simulink model "vehicle_dynamics_fullcar"  (R2012b)
settings: Solver=ode4  StartTime=0.0  StopTime=20  FixedStep=0.001  RelTol=1e-3
model workspace (MAT data in the model file):
  x0 = [0; 0; 0; 0; 0; 0; 0; 0; 0; 0; 0; 0; 0; 0]
undefined symbols (not defined in the file): CarBody, Suspension, Wheel
settings Model: Creator=vismso  LastModifiedBy=vikafla
settings DataIOCC: SaveFinalState=on  SignalLoggingSaveFormat=ModelDataLogs  SaveOutput=off  SaveTime=off
settings OptimizationCC: InlineParams=on
settings DebuggingCC: FcnCallInpInsideContextMsg=UseLocalSettings  StrictBusMsg=Warning
settings SFSimCC: SimParseCustomCode=off
settings GRTTargetCC: CombineOutputUpdateFcns=off  GRTInterface=on

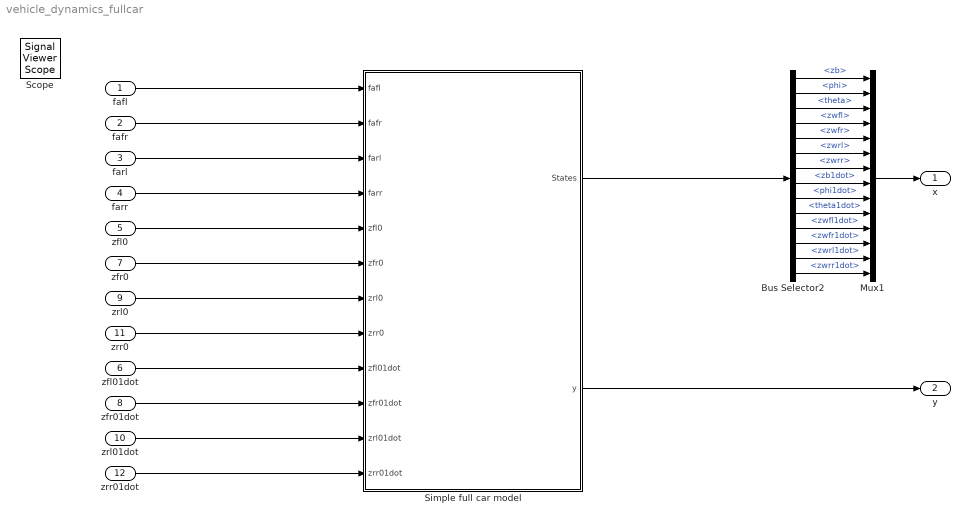
== system vehicle_dynamics_fullcar ==
  fafl : Inport
  fafr : Inport  Port=2
  farl : Inport  Port=3
  farr : Inport  Port=4
  zfl0 : Inport  Port=5
  zfl01dot : Inport  Port=6
  zfr0 : Inport  Port=7
  zfr01dot : Inport  Port=8
  zrl0 : Inport  Port=9
  zrl01dot : Inport  Port=10
  zrr0 : Inport  Port=11
  zrr01dot : Inport  Port=12
  Bus Selector2 : BusSelector  OutputSignals=zb,phi,theta,zwfl,zwfr,zwrl,zwrr,zb1dot,phi1dot,theta1dot,zwfl1dot,zwfr1dot,zwrl1dot,zwrr1dot
  Mux1 : Mux  Inputs=14
  Simple full car model : Subsystem  mask{mb=CarBody.Mass, mw=Wheel.Mass, Ibxx=CarBody.InertiaTensor(1,1), Ibyy=CarBody.InertiaTensor(2,2), lf=Suspension.MountPointFL(1), lr=-Suspension.MountPointRL(1), hf=Suspension.MountPointFL(3), hr=Suspension.MountPointRL(3), d=Suspension.MountPointFL(1)-Suspension.MountPointRL(1), tw=Suspension.MountPointFL(2)-Suspension.MountPointFR(2), r0=Wheel.UnloadedRadius, g=9.81, l0f=Suspension.SpringFreeLengthFL, l0r=Suspension.SpringFreeLengthRL, crbf=Suspension.FrontRollbarStiffness, crbr=Suspension.RearRollbarStiffness, cf=interp1(Suspension.SpringStiffnessLookUpFL(1,:).',Suspension.SpringStiffnessLookUpFL(2,:).',1,'linear','extrap'), cr=interp1(Suspension.SpringStiffnessLookUpRL(1,:).',Suspension.SpringStiffnessLookUpRL(2,:).',1,'linear','extrap'), df=5*interp1(Suspension.DamperCushioningLookUpFL(1,:).',Suspension.DamperCushioningLookUpFL(2,:).',1,'linear','extrap'), dr=7*interp1(Suspension.DamperCushioningLookUpRL(1,:).',Suspension.DamperCushioningLookUpRL(2,:).',1,'linear','extrap'), cw=Wheel.TireStiffness, dw=Wheel.TireDamping}
      mask prompts: mb "Vehicle body mass [kg]"; mw "Wheel mass [kg]"; Ibxx "Body inertia Ixx [kg m^2]"; Ibyy "Body inertia Iyy [kg m^2]"; lf "Distance from COG to front axle [m]"; lr "Distance from COG to rear axle [m]"; hf "Height of front damper mount points over COG [m]"; hr "Height of rear damper mount points over COG [m]"; d "Wheelbase [m]"; tw "Track width"; r0 "Unloaded tire radius [m]"; g "Gravity [m/s^2]"; l0f "Free length of front springs [m]"; l0r "Free length of rear springs [m]"; crbf "Front rollbar stiffness [N/m]"; crbr "Rear rollbar stiffness [N/m]"; cf "Front spring stiffness [N/m]"; cr "Rear spring stiffness [N/m]"; df "Front damper cushioning [Ns/m]"; dr "Rear damper cushioning [Ns/m]"; cw "Tire stiffness [N/m]"; dw "Tire damper cushioning [Ns/m]"
  x : Outport
  y : Outport  Port=2
  Scope : SignalViewerScope  IOType=viewer  ZoomMode=yonly  RefreshTime=0.035000
  wires:
  fafl/1 -> Simple full car model/1(fafl)
  fafr/1 -> Simple full car model/2(fafr)
  Simple full car model/2(y) -> y/1
  zfl0/1 -> Simple full car model/5(zfl0)
  farl/1 -> Simple full car model/3(farl)
  farr/1 -> Simple full car model/4(farr)
  zfr0/1 -> Simple full car model/6(zfr0)
  zrl0/1 -> Simple full car model/7(zrl0)
  zrr0/1 -> Simple full car model/8(zrr0)
  zfl01dot/1 -> Simple full car model/9(zfl01dot)
  zfr01dot/1 -> Simple full car model/10(zfr01dot)
  zrl01dot/1 -> Simple full car model/11(zrl01dot)
  zrr01dot/1 -> Simple full car model/12(zrr01dot)
  Simple full car model/1(States) -> Bus Selector2/1
  Bus Selector2/1 -> Mux1/1  "<zb>"
  Bus Selector2/2 -> Mux1/2  "<phi>"
  Bus Selector2/3 -> Mux1/3  "<theta>"
  Bus Selector2/4 -> Mux1/4  "<zwfl>"
  Bus Selector2/5 -> Mux1/5  "<zwfr>"
  Bus Selector2/6 -> Mux1/6  "<zwrl>"
  Bus Selector2/7 -> Mux1/7  "<zwrr>"
  Bus Selector2/8 -> Mux1/8  "<zb1dot>"
  Bus Selector2/9 -> Mux1/9  "<phi1dot>"
  Bus Selector2/10 -> Mux1/10  "<theta1dot>"
  Bus Selector2/11 -> Mux1/11  "<zwfl1dot>"
  Bus Selector2/12 -> Mux1/12  "<zwfr1dot>"
  Bus Selector2/13 -> Mux1/13  "<zwrl1dot>"
  Bus Selector2/14 -> Mux1/14  "<zwrr1dot>"
  Mux1/1 -> x/1

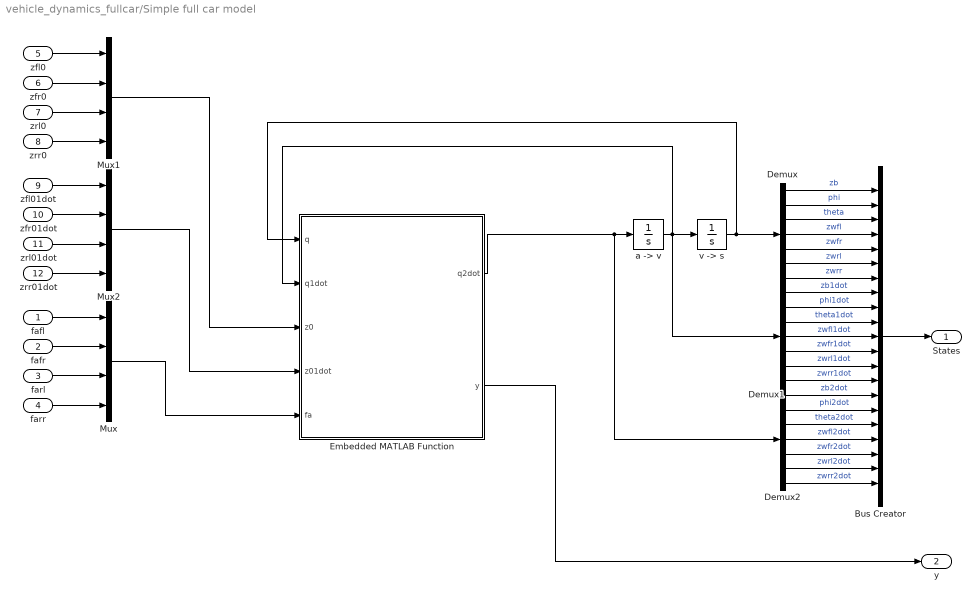
== system vehicle_dynamics_fullcar/Simple full car model ==
  fafl : Inport
  fafr : Inport  Port=2
  farl : Inport  Port=3
  farr : Inport  Port=4
  zfl0 : Inport  Port=5
  zfr0 : Inport  Port=6
  zrl0 : Inport  Port=7
  zrr0 : Inport  Port=8
  zfl01dot : Inport  Port=9
  zfr01dot : Inport  Port=10
  zrl01dot : Inport  Port=11
  zrr01dot : Inport  Port=12
  Bus Creator : BusCreator  Inputs=21
  Demux : Demux  Outputs=7
  Demux1 : Demux  Outputs=7
  Demux2 : Demux  Outputs=7
  Embedded MATLAB Function : MATLAB Function  TreatAsAtomicUnit=on
  Mux : Mux
  Mux1 : Mux
  Mux2 : Mux
  "a -> v" : Integrator  InitialCondition=x0(8:14)
  "v -> s" : Integrator  InitialCondition=x0(1:7)
  States : Outport
  y : Outport  Port=2
  wires:
  "a -> v"/1 -> "v -> s"/1, Embedded MATLAB Function/2(q1dot), Demux1/1
  Embedded MATLAB Function/1(q2dot) -> "a -> v"/1, Demux2/1
  "v -> s"/1 -> Embedded MATLAB Function/1(q), Demux/1
  fafl/1 -> Mux/1
  fafr/1 -> Mux/2
  farl/1 -> Mux/3
  farr/1 -> Mux/4
  Mux/1 -> Embedded MATLAB Function/5(fa)
  zfl0/1 -> Mux1/1
  zfr0/1 -> Mux1/2
  zrl0/1 -> Mux1/3
  zrr0/1 -> Mux1/4
  zfl01dot/1 -> Mux2/1
  zfr01dot/1 -> Mux2/2
  zrl01dot/1 -> Mux2/3
  zrr01dot/1 -> Mux2/4
  Mux1/1 -> Embedded MATLAB Function/3(z0)
  Mux2/1 -> Embedded MATLAB Function/4(z01dot)
  Demux/1 -> Bus Creator/1  "zb"
  Demux/2 -> Bus Creator/2  "phi"
  Demux/3 -> Bus Creator/3  "theta"
  Demux/4 -> Bus Creator/4  "zwfl"
  Demux/5 -> Bus Creator/5  "zwfr"
  Demux/6 -> Bus Creator/6  "zwrl"
  Demux/7 -> Bus Creator/7  "zwrr"
  Demux1/1 -> Bus Creator/8  "zb1dot"
  Demux1/2 -> Bus Creator/9  "phi1dot"
  Demux1/3 -> Bus Creator/10  "theta1dot"
  Demux1/4 -> Bus Creator/11  "zwfl1dot"
  Demux1/5 -> Bus Creator/12  "zwfr1dot"
  Demux1/6 -> Bus Creator/13  "zwrl1dot"
  Demux1/7 -> Bus Creator/14  "zwrr1dot"
  Demux2/1 -> Bus Creator/15  "zb2dot"
  Demux2/2 -> Bus Creator/16  "phi2dot"
  Demux2/3 -> Bus Creator/17  "theta2dot"
  Demux2/4 -> Bus Creator/18  "zwfl2dot"
  Demux2/5 -> Bus Creator/19  "zwfr2dot"
  Demux2/6 -> Bus Creator/20  "zwrl2dot"
  Demux2/7 -> Bus Creator/21  "zwrr2dot"
  Bus Creator/1 -> States/1
  Embedded MATLAB Function/2(y) -> y/1

== matlab function vehicle_dynamics_fullcar/Simple full car model/Embedded MATLAB Function ==
  data: q input; q2dot output size=7; q1dot input; z0 input; z01dot input; fa input; y output; g parameter; Ibyy parameter; Ibxx parameter; mb parameter; mw parameter; lf parameter; lr parameter; tw parameter; l0f parameter; l0r parameter; hf parameter; hr parameter; r0 parameter; cf parameter; df parameter; cr parameter; dr parameter; crbf parameter; crbr parameter; cw parameter; dw parameter
function [q2dot, y] = vehicle_dynamics(q,q1dot,z0, z01dot, fa, g, Ibyy, Ibxx, mb, mw, lf, lr, tw, l0f, l0r, hf, hr, r0, cf, df, cr, dr, crbf, crbr, cw, dw)
%#eml
%Parameter
b = tw/2;

zb = q(1);
phi = q(2);
theta = q(3);
zwfl = q(4);
zwfr = q(5);
zwrl = q(6);
zwrr = q(7);

zb1dot = q1dot(1);
phi1dot = q1dot(2);
theta1dot = q1dot(3);
zwfl1dot = q1dot(4);
zwfr1dot = q1dot(5);
zwrl1dot = q1dot(6);
zwrr1dot = q1dot(7);

zfl0 = z0(1);
zfr0 = z0(2);
zrl0 = z0(3);
zrr0 = z0(4);

zfl01dot = z01dot(1);
zfr01dot = z01dot(2);
zrl01dot = z01dot(3);
zrr01dot = z01dot(4);

fafl = fa(1);
fafr = fa(2);
farl = fa(3);
farr = fa(4);

% Body corner point positions
zbfl = zb-theta*lf+phi*b+hf;
zbfr = zb-theta*lf-phi*b+hf;
zbrl = zb+theta*lf+phi*b+hr;
zbrr = zb+theta*lf-phi*b+hr;

% Body corner point velocities
zbfl1dot = zb1dot-theta1dot*lf+phi1dot*b;
zbfr1dot = zb1dot-theta1dot*lf-phi1dot*b;
zbrl1dot = zb1dot+theta1dot*lf+phi1dot*b;
zbrr1dot = zb1dot+theta1dot*lf-phi1dot*b;

% Spring damper forces
FDfl = cf*(zwfl-zbfl+l0f)+df*(zwfl1dot-zbfl1dot)+fafl;
FDfr = cf*(zwfr-zbfr+l0f)+df*(zwfr1dot-zbfr1dot)+fafr;
FDrl = cr*(zwrl-zbrl+l0r)+dr*(zwrl1dot-zbrl1dot)+farl;
FDrr = cr*(zwrr-zbrr+l0r)+dr*(zwrr1dot-zbrr1dot)+farr;

%Roll bar forces

FRf = crbf*(zwfr-zwfl);
FRr = crbr*(zwrr-zwrl);

% Tire forces
FTfl = cw*(zfl0-zwfl+r0)+dw*(zfl01dot-zwfl1dot);
FTfr = cw*(zfr0-zwfr+r0)+dw*(zfr01dot-zwfr1dot);
FTrl = cw*(zrl0-zwrl+r0)+dw*(zrl01dot-zwrl1dot);
FTrr = cw*(zrr0-zwrr+r0)+dw*(zrr01dot-zwrr1dot);

if(  (zwfl-zfl0-r0) > 0 ), FTfl = 0; end;
if(  (zwfr-zfr0-r0) > 0 ), FTfr = 0; end;
if(  (zwrl-zrl0-r0) > 0 ), FTrl = 0; end;
if(  (zwrr-zrr0-r0) > 0 ), FTrr = 0; end;

zb2dot = -g + 1/mb*(FDfl+FDfr+FDrl+FDrr);
phi2dot = 1/Ibxx*(b*(FDfl+FDrl-FDfr-FDrr));
theta2dot = 1/Ibyy*(lr*(FDrl+FDrr)-lf*(FDfl+FDfr));
zwfl2dot = -g + 1/mw*(-FDfl+FTfl+FRf);
zwfr2dot = -g + 1/mw*(-FDfr+FTfr-FRf);
zwrl2dot = -g + 1/mw*(-FDrl+FTrl+FRr);
zwrr2dot = -g + 1/mw*(-FDrr+FTrr-FRr);

zbfl2dot = zb2dot-theta2dot*lf+phi2dot*b;
zbfr2dot = zb2dot-theta2dot*lf-phi2dot*b;
zbrl2dot = zb2dot+theta2dot*lf+phi2dot*b;
zbrr2dot = zb2dot+theta2dot*lf-phi2dot*b;

q2dot = [zb2dot;phi2dot;theta2dot;zwfl2dot;zwfr2dot;zwrl2dot;zwrr2dot];

% zbij = [zbfl;zbfr;zbrl;zbrr;zbfl1dot;zbfr1dot;zbrl1dot;zbrr1dot; ...
%     zbfl2dot;zbfr2dot;zbrl2dot;zbrr2dot];

y = [   zwfl-zbfl;
        zwfr-zbfr;
        zwrl-zbrl;
        zwrr-zbrr;
        zwfl1dot-zbfl1dot;
        zwfr1dot-zbfr1dot;
        zwrl1dot-zbrl1dot;
        zwrr1dot-zbrr1dot;
        zbfl1dot;
        zbfr1dot;
        zbrl1dot;
        zbrr1dot;
        zbfl2dot;
        zbfr2dot;
        zbrl2dot;
        zbrr2dot;
        zwfl1dot;
        zwfr1dot;
        zwrl1dot;
        zwrr1dot;
        zwfl2dot;
        zwfr2dot;
        zwrl2dot;
        zwrr2dot;
       ];
